simulink model "TP_loop"  (R2012b)
settings: Solver=ode45  StartTime=0.0  StopTime=100  RelTol=1e-3
settings Model: Creator=m1eea_002  LastModifiedBy=m1eea_022

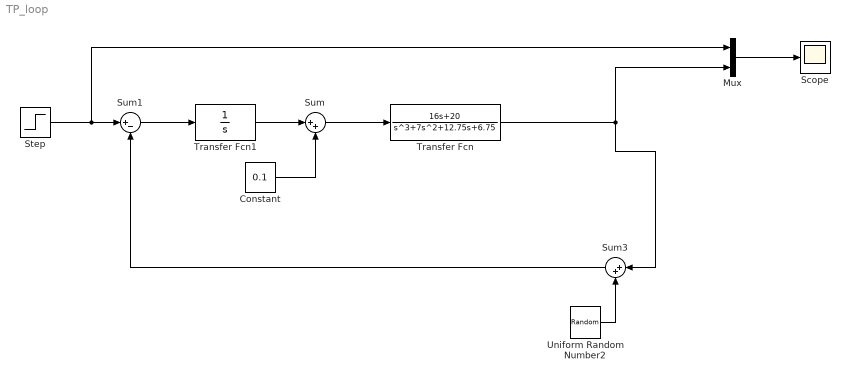
== system TP_loop ==
  Constant : Constant  Value=0.1
  Mux : Mux  Inputs=2
  Scope : Scope
  Step : Step  SampleTime=0
  Sum : Sum  Inputs=|++
  Sum1 : Sum  Inputs=|+-
  Sum3 : Sum  Inputs=|++
  Transfer Fcn : TransferFcn  Numerator=[16,20]  Denominator=[1,7,12.75,6.75]
  Transfer Fcn1 : TransferFcn  Denominator=[1 0]
  Uniform Random Number2 : UniformRandomNumber  Minimum=-0.1  Maximum=0.1  SampleTime=0.1
  wires:
  Sum/1 -> Transfer Fcn/1
  Sum3/1 -> Sum1/2
  Step/1 -> Mux/1, Sum1/1
  Mux/1 -> Scope/1
  Uniform Random Number2/1 -> Sum3/2
  Constant/1 -> Sum/2
  Transfer Fcn/1 -> Sum3/1, Mux/2
  Transfer Fcn1/1 -> Sum/1
  Sum1/1 -> Transfer Fcn1/1
